simulink model "FTCSimulation_2023a"  (R2023a)
settings: Solver=FixedStepAuto  StartTime=0.0  StopTime=SimTime  FixedStep=0.01  RelTol=1e-3
values from neighbouring files (symbols this model uses):
  g = 9.81    [aero_guid_dat.m]
  Iyy = 182.5/(Kg2slug*m2ft^2)    (= 247.436636441)    [aero_guid_dat.m]
  L = 0.0065    [aero_guid_dat.m]
undefined symbols (not defined in the file or in its folder): A_x, A_y, A_z, AF, apSampleTime, arSampleTime, B_x, B_y, B_z, c_1, c_2, c_3, c_4, C_x, C_y, C_z, CAM, Continuous, D_x, D_y, D_z, Dis, ESO, GOSELM, inertia, Ixx, Izz, K_a1, K_a2, K_a3, K_d, K_d_LQR_phi, K_d_LQR_psi, K_d_LQR_theta, K_d_LQR_x, K_d_LQR_y, K_d_LQR_z, K_p1, K_p2, K_p3, K_q_LQR_phi, K_q_LQR_psi, K_q_LQR_theta, K_q_LQR_x, K_q_LQR_y, K_q_LQR_z, lambda, m, M, Noise, SM, Time
libraries: simulink x6, ctrlSharedLib x3, eeGeneralControl x1
(part 2 of 2)

== matlab function FTCSimulation_2023a/Quadrotor Plant (Affine System Nonlinear Model)/Model ==
  data: u input; D input; X_dot output; X input
function X_dot = fcn(u,D, X)
% u = [T tau_phi tau_theta tau_psi]
% X = [x y z phi theta psi x_dot y_dot z_dot p q r]
% x=X(1), y=X(2), z=X(3), phi=X(4), theta=X(5), psi=X(6), x_dot=X(7)
% y_dot=X(8) z_dot=X(9) p=X(10) q=X(11) r=X(12)
% X_in = [z phi theta psi z_dot p q r], y_in = [z phi theta psi]

% X_dot = f(X)+g(X)u,  h=h(X)

% f(x) = [x_dot; y_dot; z_dot;
% p+q*sin(phi)*tan(theta)+r*cos(phi)*tan(theta);
% q*cos(phi)-r*sin(phi); q*sin(phi)/cos(theta)+r*cos(phi)/cos(theta);
% 0; 0; -g;(Iyy-Izz)*q*r/(Ixx); (Izz-Ixx)*p*r/(Iyy); (Ixx-Iyy)*p*q/(Izz)]

% g(X) = [zeros(6,4); (cos(phi)*sin(theta)*cos(psi)+sin(phi)*sin(psi))/m 0
% 0 0; (cos(phi)*sin(theta)*sin(psi)-sin(phi)*cos(psi))/m 0 0 0;
% (cos(phi)*cos(theta))/m 0 0 0; 0 1/Ixx 0 0; 0 0 1/Iyy 0; 0 0 0 1/Izz]

g = 9.80665; % Gravitational Acceleration [m/s^2]
m = 0.46; % Quadrotor Mass [Kg]
Ixx = 2.24e-3;
Iyy = 2.9e-3;
Izz = 5.3e-3;

f = [X(7); X(8); X(9);
X(10)+X(11)*sin(X(4))*tan(X(5))+X(12)*cos(X(4))*tan(X(5));
X(11)*cos(X(4))-X(12)*sin(X(4)); X(11)*sin(X(4))/cos(X(5))+X(12)*cos(X(4))/cos(X(5));
0+D(4); 0+D(5); -g+D(6);(Iyy-Izz)*X(11)*X(12)/(Ixx)+D(1); (Izz-Ixx)*X(10)*X(12)/(Iyy)+D(2); (Ixx-Iyy)*X(10)*X(11)/(Izz)+D(3)];

G = [zeros(6,4); (cos(X(4))*sin(X(5))*cos(X(6))+sin(X(4))*sin(X(6)))/m 0 0 0; (cos(X(4))*sin(X(5))*sin(X(6))-sin(X(4))*cos(X(6)))/m 0 0 0;
(cos(X(4))*cos(X(5)))/m 0 0 0; 0 1/Ixx 0 0; 0 0 1/Iyy 0; 0 0 0 1/Izz];

X_dot = f+G*u;

== matlab function FTCSimulation_2023a/Control/GOS-ELM-based fault estimator ==
  settings: updateMethod=DISCRETE
  data: gamma_hat output; eta input; eta_d input; x_ddot_n input; u_c input; d_hat_n input; diag_1_gamma output; Ixx parameter; Izz parameter; L parameter; c_1 parameter; c_2 parameter; c_3 parameter; c_4 parameter; Iyy parameter; lambda parameter; g parameter; m parameter
function [gamma_hat,diag_1_gamma] = fcn(eta,eta_d,x_ddot_n,u_c,d_hat_n, Ixx, Izz, L, c_1, c_2, c_3, c_4, Iyy, lambda, g, m)
persistent gamma
if isempty(gamma)
    gamma = [1; 1; 1; 1];
end
persistent gamma_f
if isempty(gamma_f)
    gamma_f = [1; 1; 1; 1];
end
persistent LL
if isempty(LL)
    LL = 100*eye(4);
end
% system
f_n = [-g;
    (Iyy-Izz)*eta_d(2)*eta_d(3)/(Ixx);
    (Izz-Ixx)*eta_d(1)*eta_d(3)/(Iyy);
    (Ixx-Iyy)*eta_d(1)*eta_d(2)/(Izz)];

g_n = [cos(eta(1))*cos(eta(2))/m cos(eta(1))*cos(eta(2))/m ...
    cos(eta(1))*cos(eta(2))/m cos(eta(1))*cos(eta(2))/m;
    L/Ixx -L/Ixx -L/Ixx L/Ixx;
    -L/Iyy -L/Iyy L/Iyy L/Iyy;
    c_1/Izz -c_2/Izz c_3/Izz -c_4/Izz];

% GOS-ELM
Delta_u = x_ddot_n-f_n-d_hat_n;
mu = (g_n*diag(u_c)).';

LL = LL/lambda-LL*mu*inv(lambda*eye(4)+mu.'*LL*mu)*mu.'*LL/lambda;
gamma = gamma +LL*mu*(Delta_u-mu.'*gamma);
gamma = min(gamma,1);
gamma = max(gamma,0.5);
gamma_f = gamma_f + 0.01/0.5*(gamma-gamma_f);
gamma_hat = gamma_f;
diag_1_gamma = diag(1./gamma_f);

== matlab function FTCSimulation_2023a/Control Allocator/RotorThrustToPWM ==
  data: T input; PWM output
function PWM = fcn(T)
a1_bar = 1.14e-4; b1_bar = 1.018e-2; c1_bar = 6.5833e-2;
a2_bar = 1.1544e-4; b2_bar = 7.7509e-3; c2_bar = 9.5961e-2;
a3_bar = 1.2605e-4; b3_bar = 9.2952e-3; c3_bar = 7.214e-2;
a4_bar = 1.3045e-4; b4_bar = 7.5567e-3; c4_bar = 8.2877e-2;

PWM1 = (-b1_bar+sqrt((b1_bar)^2-4*(a1_bar)*(c1_bar-T(1))))/(2*(a1_bar));
PWM2 = (-b2_bar+sqrt((b2_bar)^2-4*(a2_bar)*(c2_bar-T(2))))/(2*(a2_bar));
PWM3 = (-b3_bar+sqrt((b3_bar)^2-4*(a3_bar)*(c3_bar-T(3))))/(2*(a3_bar));
PWM4 = (-b4_bar+sqrt((b4_bar)^2-4*(a4_bar)*(c4_bar-T(4))))/(2*(a4_bar));

PWM = [PWM1 PWM2 PWM3 PWM4];

== matlab function FTCSimulation_2023a/Control/Feedback Linearization + LQI/State Feedback Linearization/MATLAB Function ==
  data: v_in input; u_in output; x_hat input; Ix input; Iy input; Iz input; g input; m input
function u_in = fcn(v_in, x_hat,Ix,Iy,Iz,g,m)

phi = x_hat(4);
theta = x_hat(5);
p = x_hat(10);
q = x_hat(11);
r = x_hat(12);

alpha = [(g*m)/(cos(phi)*cos(theta));
         (Iz-Iy-Ix*cos(2*phi))*q*r + 0.5*sin(2*phi)*Ix*(r^2-q^2);
         Iy*cos(phi)*tan(theta)*(2*r^2-q^2)+p*r*(Ix+Iy-Iz)+Iy*((cos(phi))^3)*tan(theta)*(q^2-r^2)+2*Iy*q*r*((sin(phi))^3)*tan(theta);
         -(Iz*q^2*sin(phi)*tan(theta)+p*q*(Ix-Iy+Iz)+Iz*((cos(phi))^2)*sin(phi)*tan(theta)*(q^2-r^2)+2*Iz*q*r*((cos(phi))^3)*tan(theta))];

beta = [m/(cos(phi)*cos(theta)) 0 0 0;
        0 Ix 0 -Ix*sin(theta);
        0 0 Iy*cos(phi) Iy*cos(theta)*sin(phi);
        0 0 -Iz*sin(phi) Iz*cos(phi)*cos(theta)];

u_in = alpha + beta*v_in;

== matlab function FTCSimulation_2023a/Desired Trajectory ==
  data: x_d output; y_d output; z_d output; psi_d output; t input; SimulationMode input
function [x_d,y_d,z_d,psi_d] = fcn(t,SimulationMode)
if SimulationMode == 1 %Tracking
    if t<10
        x_d =0;
        y_d =0 ;
        z_d =0;
        psi_d = 0;
    elseif t>=10 && t<30
        x_d =0;
        y_d =0 ;
        z_d =0.7;
        psi_d = 0;
    elseif t>=30 && t<50
        x_d =-(t-30)/20;
        y_d =0 ;
        z_d =0.7;
        psi_d = 0;
    elseif t>=50 && t<55
        x_d =-1;
        y_d =0 ;
        z_d =0.7;
        psi_d = 0;
    elseif t>=55 && t<65
        x_d =-1;
        y_d = 0;
        z_d =0.05*(t-55)+0.7;  
        psi_d = 0;
    elseif t>=65 && t<70
        x_d =-1;
        y_d = 0;
        z_d =1.2;
        psi_d = 0;
    elseif t>=70 && t<90
        x_d =-1-0.5*sin(pi*(t-70)/20);
        y_d = -(t-70)/20;
        z_d =1.2;
        psi_d = 0;
    elseif t>=90 && t<95
        x_d =-1;
        y_d = -1;
        z_d =1.2;
        psi_d = 0;
    elseif t>=95 && t<105
        x_d =-1;
        y_d = -1;
        z_d =1.2-0.05*(t-95);
        psi_d = 0;
    elseif t>=105 && t<110
        x_d =-1;
        y_d = -1;
        z_d =0.7;
        psi_d = 0;
    elseif t>=110 && t<130
        x_d =(t-110)/20-1;
        y_d = -1;
        z_d =0.7;
        psi_d = 0;
    elseif t>=130 && t<135
        x_d =0;
        y_d =-1 ;
        z_d =0.7;
        psi_d = 0;
    elseif t>=135 && t<145
        x_d =0;
        y_d =-1 ;
        z_d =0.05*(t-135)+0.7;
        psi_d = 0;
    elseif t>=145 && t<150
        x_d =0;
        y_d =-1 ;
        z_d =1.2;
        psi_d = 0;
    elseif t>=150 && t<170
        x_d =0.5*sin(pi*(t-150)/20);
        y_d = (t-170)/20;
        z_d =1.2;
        psi_d = 0;
    elseif t>=170 && t<175
        x_d =0;
        y_d = 0;
        z_d =1.2;
        psi_d = 0;
    elseif t>=175 && t<185
        x_d =0;
        y_d = 0;
        z_d =1.2-0.05*(t-175);
        psi_d = 0;
    else 
        x_d =0;
        y_d = 0;
        z_d =0.7;
        psi_d = 0;
    end
elseif SimulationMode == 2 % Uncertainty
     if t<10
        x_d =0;
        y_d =0 ;
        z_d =0;
        psi_d = 0;
    elseif t>=10 && t<20
        x_d =0;
        y_d =0 ;
        z_d =3;
        psi_d = 0;
    elseif t>=20 && t<30
        x_d =3;
        y_d =0 ;
        z_d =3;
        psi_d = 0;  
    elseif t>=30 && t<40
        x_d =3;
        y_d =3 ;
        z_d =3;
        psi_d = 0;
    elseif t>=40 && t<50
        x_d =3;
        y_d =3 ;
        z_d =3;
        psi_d = 0.1*(t-40);
%         psi_d = 0;
    elseif t>=50 && t<60
        x_d =3;
        y_d =3 ;
        z_d =6;
        psi_d = 1;
%         psi_d = 0;
    elseif t>=60 && t<70
        x_d =6;
        y_d =3 ;
        z_d =6;
      psi_d = 1;
%         psi_d = 0;
     else
        x_d =6;
        y_d =6 ;
        z_d =6;
      psi_d = 1;
%         psi_d = 0;
     end
else % Mode 3 for 3d graphical simulation
    if t<35
        x_d =2*t;
        y_d =0 ;
        z_d =3;
        psi_d = 0;
    elseif t>=35 && t<50
        x_d =0.4*(t-35)+70;
        y_d =-(t-35);
        z_d = 4;
        psi_d = -0.1*(t-35);
    elseif t>=50 && t<58
        x_d =76;
        y_d =-15;
        z_d = 4;
        psi_d = -1.5;
     else
        x_d =76;
        y_d =-15;
        z_d = 0;
        psi_d = -1.5;
     end
end

== matlab function FTCSimulation_2023a/Disturbance ==
  data: Dis input; D output; t input
function D = fcn(Dis, t)
if Dis == 1
    D = [0.1*sin(pi*t/2);
         0.05*sin(pi*t/3+pi/5);
         0.02*cos(pi*t);
         0;
         0.1;
         0.5*sin(10*pi*t+pi/10)];
else
    D = zeros(6,1);
end

== matlab function FTCSimulation_2023a/Quadrotor Plant (Affine System Nonlinear Model)/MotorThrustMoment/Actuator Fault ==
  data: AF input; u_c input; u output; t input
function u = fcn(AF,u_c, t)
if AF == 1
    if t<50
        u = u_c;
    elseif t>=50 && t<70
        u = diag([0.8,1,1,1])*u_c;
    else
        u = diag([0.8,1,0.7,1])*u_c;
    end
else
    u = u_c;
end
